simulink model "myadrc"  (R2017b)
settings: Solver=VariableStepAuto  StartTime=0.0  StopTime=10.0  RelTol=1e-3
settings Model: Creator=apple  LastModifiedBy=apple

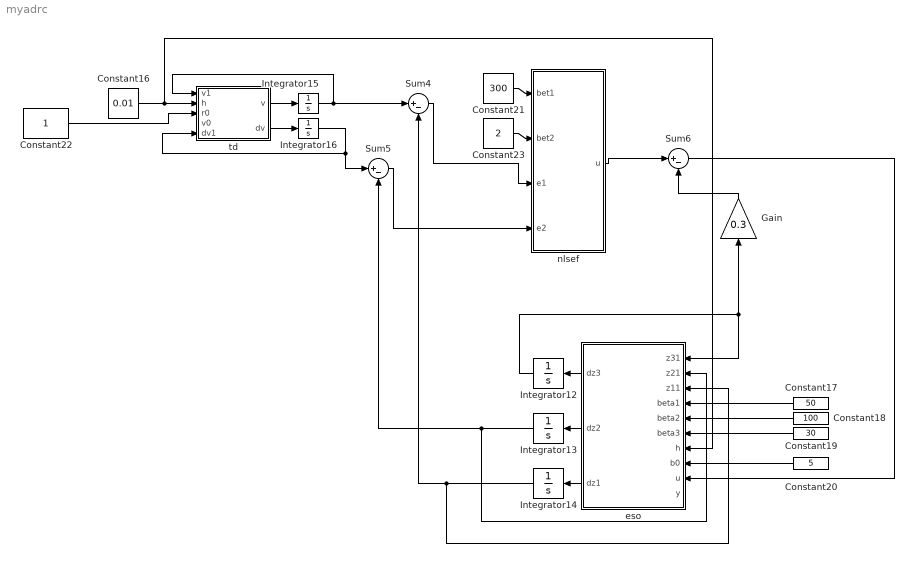
== system myadrc ==
  Constant16 : Constant  Value=0.01
  Constant17 : Constant  Value=50
  Constant18 : Constant  Value=100
  Constant19 : Constant  Value=30
  Constant20 : Constant  Value=5
  Constant21 : Constant  Value=300
  Constant22 : Constant
  Constant23 : Constant  Value=2
  Gain : Gain  Gain=0.3
  Integrator{12..16} (5 alike) : Integrator
  Sum4 : Sum  Inputs=|+-
  Sum5 : Sum  Inputs=|+-
  Sum6 : Sum  Inputs=|+-
  eso : MATLAB Function  TreatAsAtomicUnit=on
  nlsef : MATLAB Function  TreatAsAtomicUnit=on
  td : MATLAB Function  TreatAsAtomicUnit=on
  wires:
  Constant21/1 -> nlsef/1(bet1)
  Constant18/1 -> eso/5(beta2)
  eso/2(dz2) -> Integrator13/1
  Sum6/1 -> eso/9(u)
  Sum5/1 -> nlsef/4(e2)
  Integrator16/1 -> Sum5/1, td/5(dv1)
  td/1(v) -> Integrator15/1
  Constant22/1 -> td/3(r0)
  td/2(dv) -> Integrator16/1
  Constant17/1 -> eso/4(beta1)
  eso/1(dz3) -> Integrator12/1
  nlsef/1(u) -> Sum6/1
  Integrator12/1 -> eso/1(z31), Gain/1
  Constant23/1 -> nlsef/2(bet2)
  Sum4/1 -> nlsef/3(e1)
  eso/3(dz1) -> Integrator14/1
  Integrator14/1 -> Sum4/2, eso/3(z11)
  Constant20/1 -> eso/8(b0)
  Constant16/1 -> eso/7(h), td/2(h)
  Gain/1 -> Sum6/2
  Constant19/1 -> eso/6(beta3)
  Integrator13/1 -> Sum5/2, eso/2(z21)
  Integrator15/1 -> Sum4/1, td/1(v1)

== matlab function myadrc/td ==
  data: v1 input; h input; r0 input; v0 input; dv1 input; v output; dv output
function [v,dv] = td(v1,h,r0,v0,dv1)

%fh = fhan(v1 - v0,dv1,r0,h)
d = r0 * h * h;
a0 = h * dv1;
y = v1 - v0 + a0;
a1 = sqrt(d * (d + 8 * abs(y)));
a2 = a0 + sign(y) * (a1 - d)/2;
a = (a0 + y -a2) * (sign(y + d) - sign(y - d))/2 + a2;
fh = -r0 * (a/d - sign(a)) * (sign(a + d) - sign(a - d))/2 - r0 * sign(a);

v = dv1;
dv = fh;
%v = v1 + h * dv1;
%dv = dv1 + h * fh;
end

== matlab function myadrc/nlsef ==
  data: bet1 input; bet2 input; e1 input; u output; e2 input
function u = nlsef(bet1,bet2,e1,e2)

a1 = 0.5;
a2 = 0.75;
delta1 = 0.001;
delta2 = 0.001;
u = bet1 * fal(e1,a1,delta1) + bet2 * fal(e2,a2,delta2);
end

function fe = fal(error,pow,threshold)
if abs(error) > threshold
    fe = (abs(error))^pow * sign(error);
else
    fe = error * threshold^(pow - 1);
end
end

== matlab function myadrc/eso ==
  data: dz3 output; dz2 output; z31 input; z21 input; z11 input; beta1 input; beta2 input; beta3 input; h input; b0 input; dz1 output; u input; y input
function [dz3,dz2,dz1] = eso(z31,z21,z11,beta1,beta2,beta3,h,b0,u,y)

%ts = 0.001;
e = z11 - y;
dz1 = z21 - beta1 * e;
dz2 = z31 - beta2 * fal(e,0.5,h) + b0 * u;
dz3 = -beta3 * fal(e,0.25,h);

end

function fe = fal(error,pow,threshold)
if abs(error) > threshold
    fe = (abs(error))^pow * sign(error);
else
    fe = error * threshold^(pow - 1);
end
end
